simulink model "cubesat2"  (Simulink 7.9)
settings: Solver=ode3  StartTime=0.0  StopTime=4  FixedStep=Tsample  RelTol=1e-3
values from neighbouring files (symbols this model uses):
  Iwheel = 1    [cubesat2_variables.m]
  Tsample = .001    (= 0.001)    [cubesat2_variables.m]
libraries: aerolibutil x5, aerolibtransform2 x1
settings Model: Creator=Dmitriy  LastModifiedBy=Dmitriy

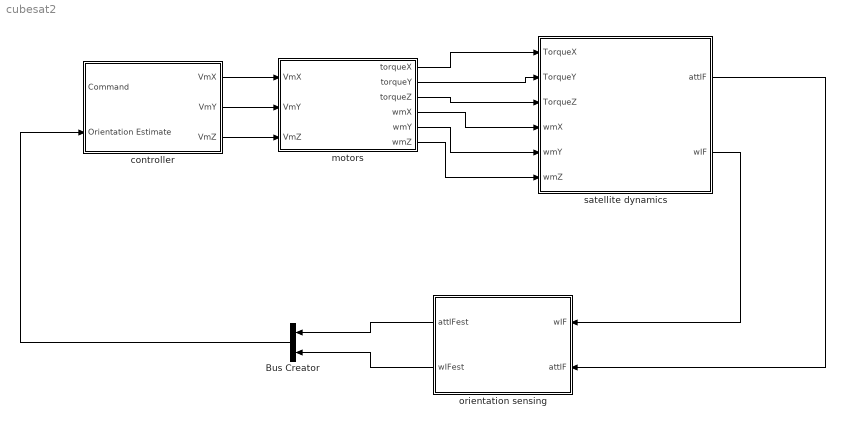
== system cubesat2 ==
  Bus Creator : BusCreator  Inputs=2
  controller : Subsystem
  motors : Subsystem
  orientation sensing : Subsystem
  satellite dynamics : Subsystem
  wires:
  motors/1(torqueX) -> satellite dynamics/1(TorqueX)
  motors/2(torqueY) -> satellite dynamics/2(TorqueY)
  motors/3(torqueZ) -> satellite dynamics/3(TorqueZ)
  controller/1(VmX) -> motors/1(VmX)
  controller/2(VmY) -> motors/2(VmY)
  controller/3(VmZ) -> motors/3(VmZ)
  motors/4(wmX) -> satellite dynamics/4(wmX)
  motors/5(wmY) -> satellite dynamics/5(wmY)
  motors/6(wmZ) -> satellite dynamics/6(wmZ)
  satellite dynamics/1(attIF) -> orientation sensing/2(attIF)
  satellite dynamics/2(wIF) -> orientation sensing/1(wIF)
  orientation sensing/1(attIFest) -> Bus Creator/1
  orientation sensing/2(wIFest) -> Bus Creator/2
  Bus Creator/1 -> controller/2(Orientation Estimate)

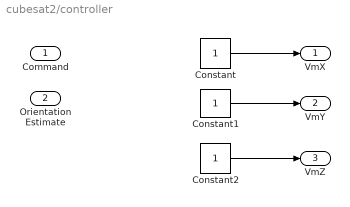
== system cubesat2/controller ==
  Command : Inport
  Orientation Estimate : Inport  Port=2
  Constant : Constant
  Constant1 : Constant
  Constant2 : Constant
  VmX : Outport
  VmY : Outport  Port=2
  VmZ : Outport  Port=3
  wires:
  Constant/1 -> VmX/1
  Constant1/1 -> VmY/1
  Constant2/1 -> VmZ/1

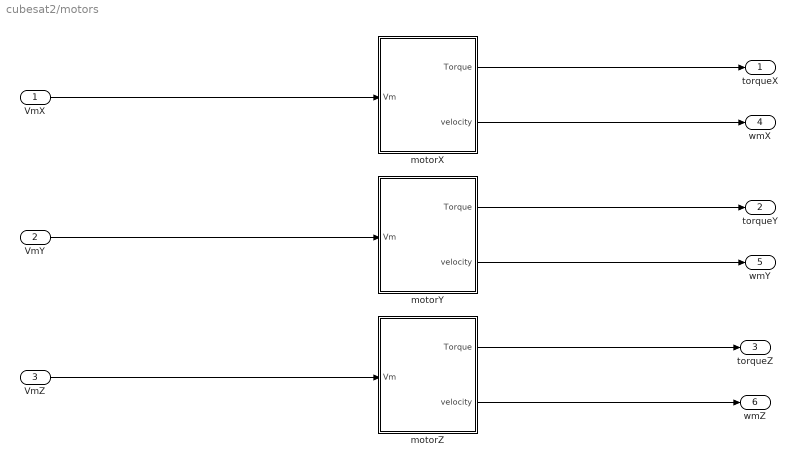
== system cubesat2/motors ==
  VmX : Inport
  VmY : Inport  Port=2
  VmZ : Inport  Port=3
  motorX : Subsystem
  motorY : Subsystem
  motorZ : Subsystem
  torqueX : Outport
  torqueY : Outport  Port=2
  torqueZ : Outport  Port=3
  wmX : Outport  Port=4
  wmY : Outport  Port=5
  wmZ : Outport  Port=6
  wires:
  VmX/1 -> motorX/1(Vm)
  motorX/1(Torque) -> torqueX/1
  motorX/2(velocity) -> wmX/1
  motorY/1(Torque) -> torqueY/1
  motorY/2(velocity) -> wmY/1
  VmY/1 -> motorY/1(Vm)
  VmZ/1 -> motorZ/1(Vm)
  motorZ/1(Torque) -> torqueZ/1
  motorZ/2(velocity) -> wmZ/1

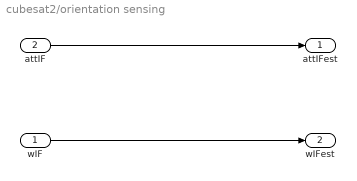
== system cubesat2/orientation sensing ==
  wIF : Inport
  attIF : Inport  Port=2
  attIFest : Outport
  wIFest : Outport  Port=2
  wires:
  attIF/1 -> attIFest/1
  wIF/1 -> wIFest/1

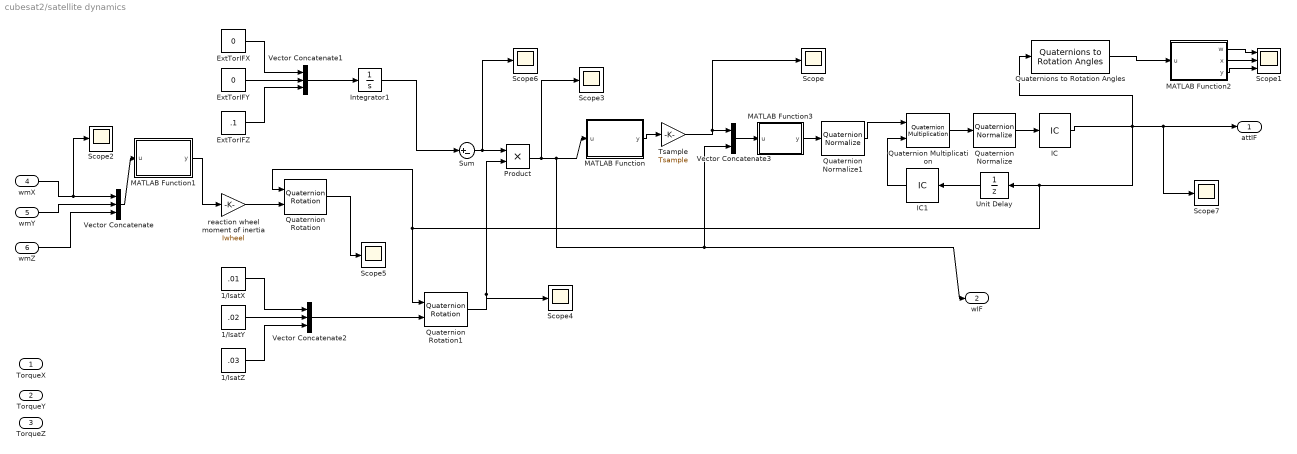
== system cubesat2/satellite dynamics ==
  TorqueX : Inport
  TorqueY : Inport  Port=2
  TorqueZ : Inport  Port=3
  wmX : Inport  Port=4
  wmY : Inport  Port=5
  wmZ : Inport  Port=6
  1/IsatX : Constant  Value=.01
  1/IsatY : Constant  Value=.02
  1/IsatZ : Constant  Value=.03
  ExtTorIFX : Constant  Value=0
  ExtTorIFY : Constant  Value=0
  ExtTorIFZ : Constant  Value=.1
  IC : InitialCondition  Value=[0 0 0 1]
  IC1 : InitialCondition  Value=[0 0 0 1]
  Integrator1 : Integrator  InitialCondition=.01
  MATLAB Function : MATLAB Function  TreatAsAtomicUnit=on
  MATLAB Function1 : MATLAB Function  TreatAsAtomicUnit=on
  MATLAB Function2 : MATLAB Function  TreatAsAtomicUnit=on
  MATLAB Function3 : MATLAB Function  TreatAsAtomicUnit=on
  Product : Product  RndMeth=Zero
  Quaternion Multiplication : aerolibutil/Quaternion Multiplication
  Quaternion Normalize : aerolibutil/Quaternion Normalize
  Quaternion Normalize1 : aerolibutil/Quaternion Normalize
  Quaternion Rotation : aerolibutil/Quaternion Rotation
  Quaternion Rotation1 : aerolibutil/Quaternion Rotation
  Quaternions to Rotation Angles : aerolibtransform2/Quaternions to Rotation Angles  rotationOrder=ZYX
  Scope{,2..7} (7 alike) : Scope
      Scope2 settings: SaveName=ScopeData2
      Scope3 settings: SaveName=ScopeData3
      Scope4 settings: SaveName=ScopeData4
      Scope5 settings: TimeRange=0.2850574712643679  YMin=-1.268781302170286  YMax=0.08347245409014814  SaveName=ScopeData5
      Scope6 settings: SaveName=ScopeData6
      Scope7 settings: SaveName=ScopeData7
  Scope1 : Scope  NumInputPorts=3
      settings: YMin=-5~-5~-5  YMax=5~5~5
  Sum : Sum  Inputs=|+-
  Tsample : Gain  Gain=Tsample
  Unit Delay : UnitDelay  SampleTime=-1
  Vector Concatenate : Concatenate  NumInputs=3
  Vector Concatenate1 : Concatenate  NumInputs=3
  Vector Concatenate2 : Concatenate  NumInputs=3
  Vector Concatenate3 : Concatenate
  reaction wheel moment of inertia : Gain  Gain=Iwheel
  attIF : Outport
  wIF : Outport  Port=2
  wires:
  wmX/1 -> Vector Concatenate/1, Scope2/1
  wmY/1 -> Vector Concatenate/2
  wmZ/1 -> Vector Concatenate/3
  Vector Concatenate/1 -> MATLAB Function1/1(u)
  reaction wheel moment of inertia/1 -> Quaternion Rotation/2
  ExtTorIFX/1 -> Vector Concatenate1/1
  ExtTorIFY/1 -> Vector Concatenate1/2
  ExtTorIFZ/1 -> Vector Concatenate1/3
  Quaternion Rotation/1 -> Scope5/1
  1/IsatX/1 -> Vector Concatenate2/1
  1/IsatY/1 -> Vector Concatenate2/2
  1/IsatZ/1 -> Vector Concatenate2/3
  Vector Concatenate1/1 -> Integrator1/1
  Integrator1/1 -> Sum/1
  Sum/1 -> Product/1, Scope6/1
  Quaternion Rotation1/1 -> Product/2, Scope4/1
  Product/1 -> MATLAB Function/1(u), wIF/1, Vector Concatenate3/2, Scope3/1
  MATLAB Function/1(y) -> Tsample/1
  Tsample/1 -> Vector Concatenate3/1, Scope/1
  Vector Concatenate2/1 -> Quaternion Rotation1/2
  IC/1 -> Quaternions to Rotation Angles/1, Unit Delay/1, Quaternion Rotation1/1, Quaternion Rotation/1, attIF/1, Scope7/1
  MATLAB Function1/1(y) -> reaction wheel moment of inertia/1
  Quaternion Normalize/1 -> IC/1
  Quaternion Multiplication/1 -> Quaternion Normalize/1
  Quaternion Normalize1/1 -> Quaternion Multiplication/1
  MATLAB Function2/1(w) -> Scope1/1
  MATLAB Function2/2(x) -> Scope1/2
  MATLAB Function2/3(y) -> Scope1/3
  Quaternions to Rotation Angles/1 -> MATLAB Function2/1(u)
  MATLAB Function3/1(y) -> Quaternion Normalize1/1
  Vector Concatenate3/1 -> MATLAB Function3/1(u)
  Unit Delay/1 -> IC1/1
  IC1/1 -> Quaternion Multiplication/2

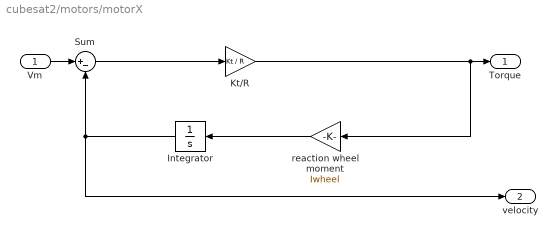
== system cubesat2/motors/motorX ==
  Vm : Inport
  Integrator : Integrator
  Kt/R : Gain  Gain=Kt / R
  Sum : Sum  Inputs=|+-
  reaction wheel moment : Gain  Gain=Iwheel
  Torque : Outport
  velocity : Outport  Port=2
  wires:
  Integrator/1 -> Sum/2, velocity/1
  Sum/1 -> Kt/R/1
  Kt/R/1 -> reaction wheel moment/1, Torque/1
  reaction wheel moment/1 -> Integrator/1
  Vm/1 -> Sum/1

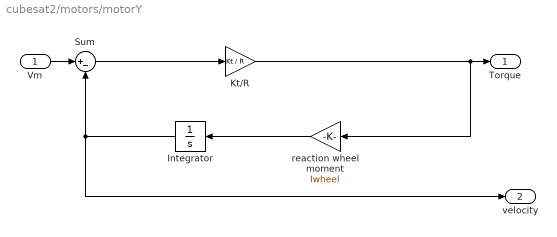
== system cubesat2/motors/motorY ==
  Vm : Inport
  Integrator : Integrator
  Kt/R : Gain  Gain=Kt / R
  Sum : Sum  Inputs=|+-
  reaction wheel moment : Gain  Gain=Iwheel
  Torque : Outport
  velocity : Outport  Port=2
  wires:
  Integrator/1 -> Sum/2, velocity/1
  Sum/1 -> Kt/R/1
  Kt/R/1 -> reaction wheel moment/1, Torque/1
  reaction wheel moment/1 -> Integrator/1
  Vm/1 -> Sum/1

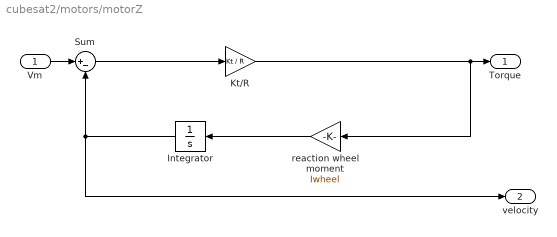
== system cubesat2/motors/motorZ ==
  Vm : Inport
  Integrator : Integrator
  Kt/R : Gain  Gain=Kt / R
  Sum : Sum  Inputs=|+-
  reaction wheel moment : Gain  Gain=Iwheel
  Torque : Outport
  velocity : Outport  Port=2
  wires:
  Integrator/1 -> Sum/2, velocity/1
  Sum/1 -> Kt/R/1
  Kt/R/1 -> reaction wheel moment/1, Torque/1
  reaction wheel moment/1 -> Integrator/1
  Vm/1 -> Sum/1

== matlab function satellite dynamics/MATLAB Function2 ==
  data: w output double; x output double; u input double; y output double
function [w,x,y] = uncat(u)
%#codegen

w = u(1);
x = u(2);
y = u(3);

== matlab function satellite dynamics/MATLAB Function ==
  data: u input double; y output double
function y = magnitude(u)
%#codegen
'product'
u
y=sqrt(sum(u.*u));

== matlab function satellite dynamics/MATLAB Function1 ==
  data: u input double; y output double
function y = fcn(u)
%#codegen
'speeds'
u
y = u;

== matlab function satellite dynamics/MATLAB Function3 ==
  data: u input double; y output double
function y = no_zero_quat(u)
%#codegen
if( sum(u==[0 0 0 0]')==4)
    y=[0 0 0 1]';
else
    y=u;
end
